simulink model "Coupled_Model_V2_C"  (R2024b)
settings: Solver=FixedStepAuto  StartTime=0.0  StopTime=20  FixedStep=0.001  RelTol=1e-3
values from neighbouring files (symbols this model uses):
  A = 2    [Setup_script_coupled_v1.m]    (also in animation_coupled_model.m; wheel_velocity_demonstrations.m)
  a = 0.8    [Setup_script_coupled_v1.m]    (also in animation_coupled_model.m; wheel_velocity_demonstrations.m)
  b = 1    [Setup_script_coupled_v1.m]    (also in animation_coupled_model.m; wheel_velocity_demonstrations.m)
  brake_bias = 0.5    [Setup_script_coupled_v1.m]    (also in animation_coupled_model.m; wheel_velocity_demonstrations.m)
  brake_torque = [0, 25, 50, 100, 125, 150, 175, 200]    [Setup_script_coupled_v1.m]    (also in animation_coupled_model.m; wheel_velocity_demonstrations.m)
  c = 0.8    [Setup_script_coupled_v1.m]    (also in animation_coupled_model.m; wheel_velocity_demonstrations.m)
  c_alpha = 30000    [Setup_script_coupled_v1.m]    (also in animation_coupled_model.m; wheel_velocity_demonstrations.m)
  C_d = 0.3    [Setup_script_coupled_v1.m]    (also in animation_coupled_model.m; wheel_velocity_demonstrations.m)
  c_sigma = 8000    [Setup_script_coupled_v1.m]    (also in animation_coupled_model.m; wheel_velocity_demonstrations.m)
  d = 0.5    [Setup_script_coupled_v1.m]    (also in animation_coupled_model.m; wheel_velocity_demonstrations.m)
  drivetrain_e = 0.8    [Setup_script_coupled_v1.m]    (also in animation_coupled_model.m; wheel_velocity_demonstrations.m)
  e = 1    [Setup_script_coupled_v1.m]    (also in animation_coupled_model.m; wheel_velocity_demonstrations.m)
  F_i_r = m_i*g-F_h    (= 327)    [Setup_script_coupled_v1.m]    (also in animation_coupled_model.m; wheel_velocity_demonstrations.m)
  F_t_f = (m_t*g*b - F_h*c)/(a+b)    (= 1889.33333333)    [Setup_script_coupled_v1.m]    (also in animation_coupled_model.m; wheel_velocity_demonstrations.m)
  F_t_r = (m_t*g*a + F_h*(b+a))/(a+b)    (= 2398)    [Setup_script_coupled_v1.m]    (also in animation_coupled_model.m; wheel_velocity_demonstrations.m)
  gr = 1    [Setup_script_coupled_v1.m]    (also in animation_coupled_model.m; wheel_velocity_demonstrations.m)
  I_pin = Izz_i + m_i*(d^2)    (= 525)    [Setup_script_coupled_v1.m]    (also in animation_coupled_model.m; wheel_velocity_demonstrations.m)
  I_wheel = 20    [Setup_script_coupled_v1.m]    (also in animation_coupled_model.m; wheel_velocity_demonstrations.m)
  Izz_t = 1000    [Setup_script_coupled_v1.m]    (also in animation_coupled_model.m; wheel_velocity_demonstrations.m)
  m_i = 100    [Setup_script_coupled_v1.m]    (also in animation_coupled_model.m; wheel_velocity_demonstrations.m)
  m_t = 400    [Setup_script_coupled_v1.m]    (also in animation_coupled_model.m; wheel_velocity_demonstrations.m)
  mu = 0.7    [Setup_script_coupled_v1.m]    (also in animation_coupled_model.m; wheel_velocity_demonstrations.m)
  peak_slip = 14*(pi/180)    (= 0.244346095279)    [Setup_script_coupled_v1.m]    (also in animation_coupled_model.m; wheel_velocity_demonstrations.m)
  r = 0.5    [Setup_script_coupled_v1.m]    (also in animation_coupled_model.m = 0.25; wheel_velocity_demonstrations.m)
  rear_braking = 0.3    [Setup_script_coupled_v1.m]    (also in animation_coupled_model.m; wheel_velocity_demonstrations.m)
  rho = 1.225    [Setup_script_coupled_v1.m]    (also in animation_coupled_model.m; wheel_velocity_demonstrations.m)
  slip_coeff = 0.3    [Setup_script_coupled_v1.m]    (also in animation_coupled_model.m; wheel_velocity_demonstrations.m)
  torque_curve = [200, 225, 300, 400, 500, 400, 350, 300, 250, 200]    [Setup_script_coupled_v1.m]    (also in animation_coupled_model.m; wheel_velocity_demonstrations.m)
  torque_omega = linspace(0, 100, length(torque_curve))    [Setup_script_coupled_v1.m]    (also in animation_coupled_model.m; wheel_velocity_demonstrations.m)
libraries: simulink x6
settings Model: Creator=lucas  LastModifiedBy=lucas
settings RTWCC: GPUComputeCapability=3.5

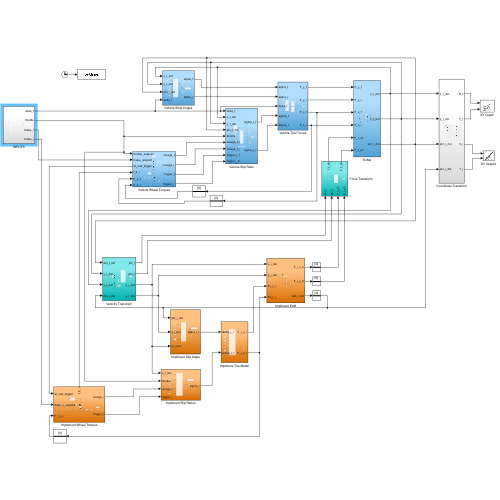
[thumbnail: Simulink's stored preview of the top-level diagram]
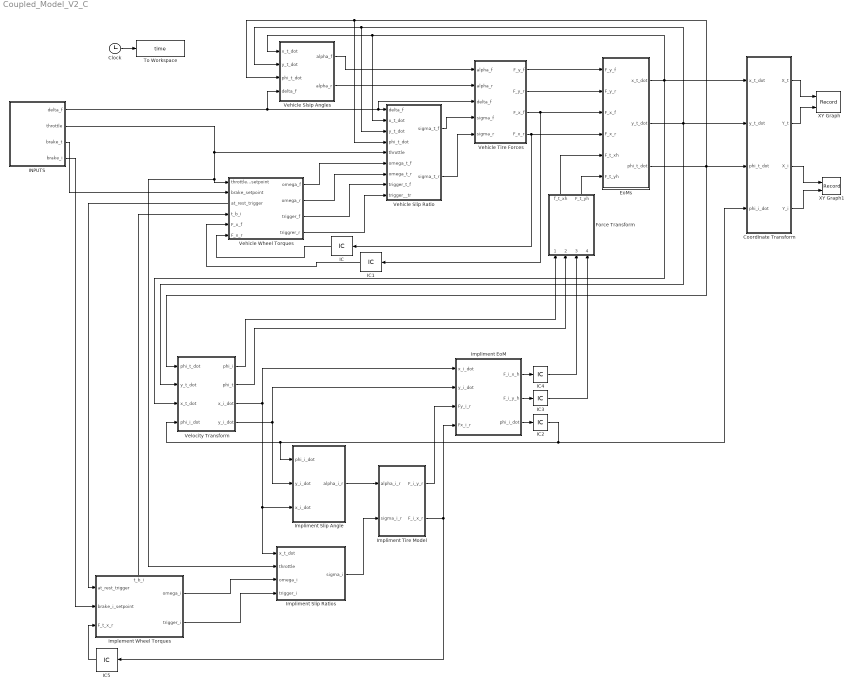
== system Coupled_Model_V2_C ==
  Clock : Clock
  Coordinate Transform : Subsystem
  EoMs : Subsystem
  Force Transform : Subsystem
  IC{,1..5} (6 alike) : InitialCondition  Value=0
  INPUTS : Subsystem
  Implement Wheel Torques : Subsystem
      settings: PortSchema="{\"entries\":[{\"content\":{\"sides\":[{\"content\":{\"connectorIds\":[\"In1\",\"In2\",\"In3\"]},\"type\":\"ConnectorPlacement.EquallySpacedRectSide\",\"uuid\":\"bbf6a9be-76e8-462d-8c03-7de9f71c826e\"},{\"content\":{\"connectorIds\":[\"Out1\",\"Out2\"],\"side\":\"RIGHT\"},\"type\":\"ConnectorPlacement.EquallySpacedRectSide\",\"uuid\":\"22c72d93-0b71-491c-9577-8b76a7679b09\"},{\"content\":{\"connectorIds\":[\"Out3\"],\"side\":\"TOP\"},\"type\":\"ConnectorPlacement.EquallySpacedRectSide\",\"uuid\":\"45839a72-84ef-4b1f-bdc9-287e587f29dc\"}]},\"type\":\"ConnectorPlacement.EquallySpacedConnector\",\"uuid\":\"4d5f4a3e-e594-4f83-8ae5-26ac09bc8c03\"}],\"packageUris\":[\"http://schema.mathworks.com/mf0/Connector/R2020b\"],\"version\":\"1.0\"}"
  Impliment EoM : Subsystem
  Impliment Slip Angle : Subsystem
  Impliment Slip Ratios : Subsystem
  Impliment Tire Model : Subsystem
  To Workspace : ToWorkspace  VariableName=time  SampleTime=-1
  Vehicle Slip Ratio : Subsystem
  Vehicle Slsip Angles : Subsystem
  Vehicle Tire Forces : Subsystem
  Vehicle Wheel Torques : Subsystem
      settings: PortSchema="{\"entries\":[{\"content\":{\"sides\":[{\"content\":{\"connectorIds\":[\"In1\",\"In2\",\"Out5\",\"In3\",\"In4\",\"In5\"]},\"type\":\"ConnectorPlacement.EquallySpacedRectSide\",\"uuid\":\"97f0ad85-6ca5-45e3-95d7-3162af9512d0\"},{\"content\":{\"connectorIds\":[\"Out1\",\"Out2\",\"Out3\",\"Out4\"],\"side\":\"RIGHT\"},\"type\":\"ConnectorPlacement.EquallySpacedRectSide\",\"uuid\":\"abd0d406-3846-4e2f-a2bd-cc2469c5c0c0\"},{\"content\":{\"side\":\"TOP\"},\"type\":\"ConnectorPlacement.EquallySpacedRectSide\",\"uuid\":\"f01a65c6-04bb-49b6-b263-3135f7c7baf2\"},{\"content\":{\"side\":\"BOTTOM\"},\"type\":\"ConnectorPlacement.EquallySpacedRectSide\",\"uuid\":\"a043eba9-81df-4422-b100-d3d245de4c1f\"}]},\"type\":\"ConnectorPlacement.EquallySpacedConnector\",\"uuid\":\"70439dd4-304f-4f7f-8815-0958974c2433\"}],\"packageUris\":[\"http://schema.mathworks.com/mf0/Connector/R2020b\"],\"version\":\"1.0\"}"
  Velocity Transform : Subsystem
  XY Graph : Record  FileSettingsInternal="{\"entries\":[{\"content\":{\"excelSettings\":{\"content\":{},\"type\":\"Streamout.ExcelSettings\"}},\"type\":\"Streamout.FileSettingStorage\",\"uuid\":\"\"}],\"packageUris\":[\"http:\\/\\/schema.mathworks.com\\/mf0\\/streamout_blocks\\/R2020a\"],\"version\":\"1.0\"}"  Layout=[1 1]  SignalsInternal="{\"entries\":[{\"content\":{\"signals\":[{\"content\":{\"blockPath\":[],\"dimensions\":[1],\"domain\":\"\",\"lineColor\":\"#139fff\",\"lineWidth\":2,\"port\":1,\"sid\":[\"\"],\"signalID\":1,\"signalName\":\"Coordinate Transform:1\"},\"type\":\"RecordBlkView.Signal\",\"uuid\":\"\"},{\"content\":{\"blockPath\":[],\"dimensions\":[1],\"domain\":\"\",\"lineColor\":\"#ff6929\",\"lineWidth\":2,\"port\":2,\"sid\":[\"\"],\"signalID\":2,\"signalName\":\"Coordinate Transform:2\"},\"type\":\"RecordBlkView.Signal\",\"uuid\":\"\"}]},\"type\":\"RecordBlkView.InputSignals\",\"uuid\":\"\"}],\"packageUris\":[\"http:\\/\\/schema.mathworks.com\\/mf0\\/streamout_blocks\\/R2020a\"],\"version\":\"1.0\"}"  VisualizationBindings="{\"xyplotplugin\":{\"info\":[{\"series\":[],\"subplotID\":1}]}}"  CompatibilityTag=XY
  XY Graph1 : Record  FileSettingsInternal="{\"entries\":[{\"content\":{\"excelSettings\":{\"content\":{},\"type\":\"Streamout.ExcelSettings\"}},\"type\":\"Streamout.FileSettingStorage\",\"uuid\":\"\"}],\"packageUris\":[\"http:\\/\\/schema.mathworks.com\\/mf0\\/streamout_blocks\\/R2020a\"],\"version\":\"1.0\"}"  Layout=[1 1]  SignalsInternal="{\"entries\":[{\"content\":{\"signals\":[{\"content\":{\"blockPath\":[],\"dimensions\":[1],\"domain\":\"\",\"lineColor\":\"#b746ff\",\"lineWidth\":2,\"port\":1,\"sid\":[\"\"],\"signalID\":1,\"signalName\":\"Coordinate Transform:3\"},\"type\":\"RecordBlkView.Signal\",\"uuid\":\"\"},{\"content\":{\"blockPath\":[],\"dimensions\":[1],\"domain\":\"\",\"lineColor\":\"#64d413\",\"lineWidth\":2,\"port\":2,\"sid\":[\"\"],\"signalID\":2,\"signalName\":\"Coordinate Transform:4\"},\"type\":\"RecordBlkView.Signal\",\"uuid\":\"\"}]},\"type\":\"RecordBlkView.InputSignals\",\"uuid\":\"\"}],\"packageUris\":[\"http:\\/\\/schema.mathworks.com\\/mf0\\/streamout_blocks\\/R2020a\"],\"version\":\"1.0\"}"  VisualizationBindings="{\"xyplotplugin\":{\"info\":[{\"series\":[],\"subplotID\":1}]}}"  CompatibilityTag=XY
  wires:
  EoMs/2(y_t_dot) -> Velocity Transform/2(y_t_dot), Coordinate Transform/2(y_t_dot), Vehicle Slip Ratio/3(y_t_dot), Vehicle Slsip Angles/2(y_t_dot)
  Vehicle Slip Ratio/1(sigma_t_f) -> Vehicle Tire Forces/4(sigma_f)
  Vehicle Slip Ratio/2(sigma_t_r) -> Vehicle Tire Forces/5(sigma_r)
  Vehicle Wheel Torques/1(omega_f) -> Vehicle Slip Ratio/6(omega_t_f)
  INPUTS/1(delta_f) -> Vehicle Slsip Angles/4(delta_f), Vehicle Tire Forces/3(delta_f), Vehicle Slip Ratio/1(delta_f)
  EoMs/3(phi_t_dot) -> Velocity Transform/1(phi_t_dot), Vehicle Slip Ratio/4(phi_t_dot), Vehicle Slsip Angles/3(phi_t_dot), Coordinate Transform/3(phi_t_dot)
  Vehicle Wheel Torques/2(omega_r) -> Vehicle Slip Ratio/7(omega_t_r)
  Vehicle Tire Forces/4(F_x_r) -> IC/1, EoMs/4(F_x_r)
  IC/1 -> Vehicle Wheel Torques/5(F_x_r)
  IC1/1 -> Vehicle Wheel Torques/4(F_x_f)
  Vehicle Tire Forces/3(F_x_f) -> IC1/1, EoMs/3(F_x_f)
  EoMs/1(x_t_dot) -> Velocity Transform/3(x_t_dot), Coordinate Transform/1(x_t_dot), Vehicle Slip Ratio/2(x_t_dot), Vehicle Slsip Angles/1(x_t_dot)
  Coordinate Transform/1(X_t) -> XY Graph/1
  Coordinate Transform/2(Y_t) -> XY Graph/2
  INPUTS/3(brake_t) -> Vehicle Wheel Torques/2(brake_setpoint)
  Vehicle Wheel Torques/3(trigger_f) -> Vehicle Slip Ratio/8(trigger_t_f)
  Vehicle Wheel Torques/4(triggrer_r) -> Vehicle Slip Ratio/9(trigger__tr)
  INPUTS/2(throttle) -> Impliment Slip Ratios/2(throttle), Vehicle Wheel Torques/1(throttle_setpoint), Vehicle Slip Ratio/5(throttle)
  Clock/1 -> To Workspace/1
  Velocity Transform/3(x_i_dot) -> Impliment Slip Angle/3(x_i_dot), Impliment Slip Ratios/1(x_t_dot), Impliment EoM/1(x_i_dot)
  Velocity Transform/4(y_i_dot) -> Impliment EoM/2(y_i_dot), Impliment Slip Angle/2(y_i_dot)
  Impliment EoM/3(phi_i_dot) -> IC2/1
  Impliment EoM/1(F_i_x_h) -> IC4/1
  Impliment EoM/2(F_i_y_h) -> IC3/1
  IC3/1 -> Force Transform/4(F_i_yh)
  IC4/1 -> Force Transform/3(F_i_xh)
  IC2/1 -> Coordinate Transform/4(phi_i_dot), Velocity Transform/4(phi_i_dot), Impliment Slip Angle/1(phi_i_dot)
  Coordinate Transform/3(X_i) -> XY Graph1/1
  Coordinate Transform/4(Y_i) -> XY Graph1/2
  Impliment Tire Model/1(F_i_y_r) -> Impliment EoM/3(Fy_i_r)
  Impliment Tire Model/2(F_i_x_r) -> IC5/1, Impliment EoM/4(Fx_i_r)
  Impliment Slip Ratios/1(sigma_i) -> Impliment Tire Model/2(sigma_i_r)
  Force Transform/2(F_t_yh) -> EoMs/6(F_t_yh)
  Force Transform/1(f_t_xh) -> EoMs/5(F_t_xh)
  Velocity Transform/2(phi_t) -> Force Transform/2(phi_t)
  Velocity Transform/1(phi_i) -> Force Transform/1(phi_i)
  Implement Wheel Torques/1(omega_i) -> Impliment Slip Ratios/3(omega_i)
  Implement Wheel Torques/2(trigger_i) -> Impliment Slip Ratios/4(trigger_i)
  Implement Wheel Torques/3(t_b_i) -> Vehicle Wheel Torques/3(t_b_i)
  INPUTS/4(brake_i) -> Implement Wheel Torques/2(brake_i_setpoint)
  IC5/1 -> Implement Wheel Torques/3(F_t_x_r)
  Vehicle Wheel Torques/5(at_rest_trigger) -> Implement Wheel Torques/1(at_rest_trigger)
  Vehicle Slsip Angles/2(alpha_r) -> Vehicle Tire Forces/2(alpha_r)
  Vehicle Slsip Angles/1(alpha_f) -> Vehicle Tire Forces/1(alpha_f)
  Vehicle Tire Forces/1(F_y_f) -> EoMs/1(F_y_f)
  Vehicle Tire Forces/2(F_y_r) -> EoMs/2(F_y_r)
  Impliment Slip Angle/1(alpha_i_r) -> Impliment Tire Model/1(alpha_i_r)

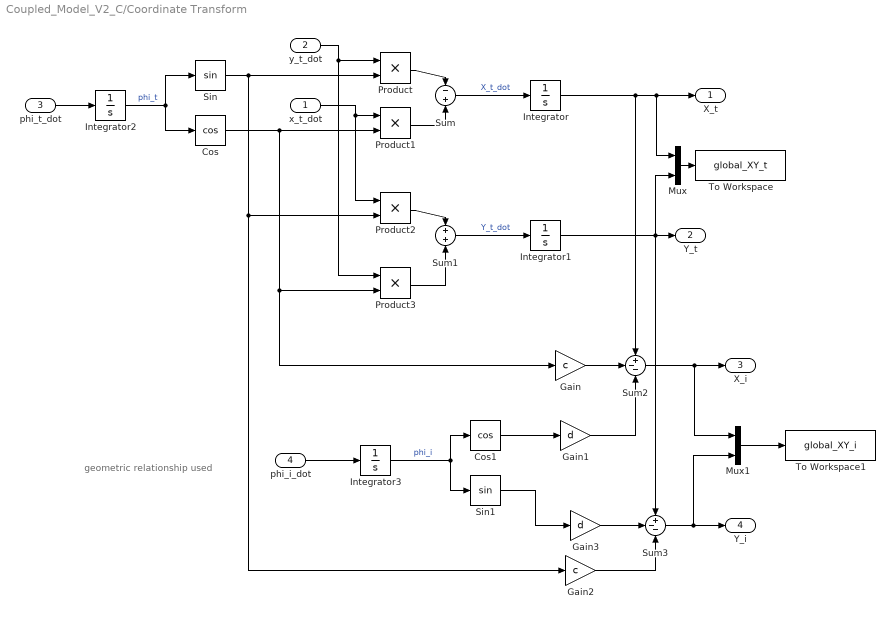
== system Coupled_Model_V2_C/Coordinate Transform ==
  note: geometric relationship used
  x_t_dot : Inport
  y_t_dot : Inport  Port=2
  phi_t_dot : Inport  Port=3
  phi_i_dot : Inport  Port=4
  Cos : Trigonometry  Operator=cos
  Cos1 : Trigonometry  Operator=cos
  Gain : Gain  Gain=c
  Gain1 : Gain  Gain=d
  Gain2 : Gain  Gain=c
  Gain3 : Gain  Gain=d
  Integrator{,1..3} (4 alike) : Integrator
  Mux : Mux  Inputs=2
  Mux1 : Mux  Inputs=2
  Product{,1..3} (4 alike) : Product
  Sin : Trigonometry
  Sin1 : Trigonometry
  Sum : Sum  Inputs=-+
  Sum1 : Sum
  Sum2 : Sum  Inputs=+--
  Sum3 : Sum  Inputs=+--
  To Workspace : ToWorkspace  VariableName=global_XY_t  SampleTime=-1
  To Workspace1 : ToWorkspace  VariableName=global_XY_i  SampleTime=-1
  X_t : Outport
  Y_t : Outport  Port=2
  X_i : Outport  Port=3
  Y_i : Outport  Port=4
  wires:
  Integrator/1 -> Sum2/1, Mux/1, X_t/1
  Integrator1/1 -> Mux/2, Y_t/1, Sum3/1
  Sum/1 -> Integrator/1  "X_t_dot"
  Sum1/1 -> Integrator1/1  "Y_t_dot"
  Sin/1 -> Product/2, Gain2/1, Product2/2
  Product/1 -> Sum/1
  Product1/1 -> Sum/2
  y_t_dot/1 -> Product/1, Product3/1
  Product2/1 -> Sum1/1
  Product3/1 -> Sum1/2
  Cos/1 -> Gain/1, Product3/2, Product1/2
  x_t_dot/1 -> Product1/1, Product2/1
  phi_t_dot/1 -> Integrator2/1
  Integrator2/1 -> Sin/1, Cos/1  "phi_t"
  Mux/1 -> To Workspace/1
  phi_i_dot/1 -> Integrator3/1
  Integrator3/1 -> Cos1/1, Sin1/1  "phi_i"
  Gain/1 -> Sum2/2
  Gain1/1 -> Sum2/3
  Cos1/1 -> Gain1/1
  Sum3/1 -> Mux1/2, Y_i/1
  Gain2/1 -> Sum3/3
  Gain3/1 -> Sum3/2
  Sin1/1 -> Gain3/1
  Mux1/1 -> To Workspace1/1
  Sum2/1 -> Mux1/1, X_i/1

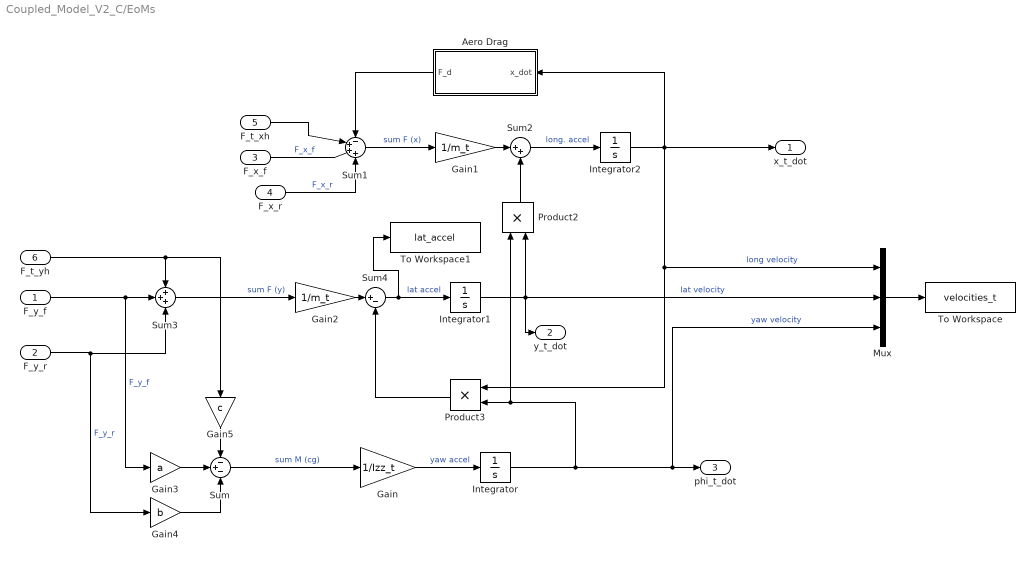
== system Coupled_Model_V2_C/EoMs ==
  F_y_f : Inport
  F_y_r : Inport  Port=2
  F_x_f : Inport  Port=3
  F_x_r : Inport  Port=4
  F_t_xh : Inport  Port=5
  F_t_yh : Inport  Port=6
  Aero Drag : Subsystem
  Gain : Gain  Gain=1/Izz_t
  Gain1 : Gain  Gain=1/m_t
  Gain2 : Gain  Gain=1/m_t
  Gain3 : Gain  Gain=a
  Gain4 : Gain  Gain=b
  Gain5 : Gain  Gain=c
  Integrator : Integrator
  Integrator1 : Integrator
  Integrator2 : Integrator
  Mux : Mux  Inputs=3
  Product2 : Product
  Product3 : Product
  Sum : Sum  Inputs=-+-
  Sum1 : Sum  Inputs=-+++
  Sum2 : Sum  Inputs=|++
  Sum3 : Sum  Inputs=+++
  Sum4 : Sum  Inputs=|+-
  To Workspace : ToWorkspace  VariableName=velocities_t  SampleTime=-1
  To Workspace1 : ToWorkspace  VariableName=lat_accel  SampleTime=-1
  x_t_dot : Outport
  y_t_dot : Outport  Port=2
  phi_t_dot : Outport  Port=3
  wires:
  Integrator1/1 -> Product2/2, Mux/2, y_t_dot/1  "lat velocity"
  Sum4/1 -> To Workspace1/1, Integrator1/1  "lat accel"
  F_y_r/1 -> Sum3/3, Gain4/1  "F_y_r"
  Sum3/1 -> Gain2/1  "sum F (y)"
  Product3/1 -> Sum4/2
  Sum/1 -> Gain/1  "sum M (cg)"
  Gain/1 -> Integrator/1  "yaw accel"
  Product2/1 -> Sum2/2
  Gain2/1 -> Sum4/1
  Gain1/1 -> Sum2/1
  Integrator/1 -> Mux/3, phi_t_dot/1, Product3/2, Product2/1  "yaw velocity"
  F_y_f/1 -> Sum3/2, Gain3/1  "F_y_f"
  Sum1/1 -> Gain1/1  "sum F (x)"
  Sum2/1 -> Integrator2/1  "long. accel"
  Integrator2/1 -> x_t_dot/1, Aero Drag/1(x_dot), Product3/1, Mux/1  "long velocity"
  Aero Drag/1(F_d) -> Sum1/1
  Mux/1 -> To Workspace/1
  Gain4/1 -> Sum/3
  Gain3/1 -> Sum/2
  Gain5/1 -> Sum/1
  F_x_r/1 -> Sum1/4  "F_x_r"
  F_x_f/1 -> Sum1/3  "F_x_f"
  F_t_xh/1 -> Sum1/2
  F_t_yh/1 -> Gain5/1, Sum3/1

== system Coupled_Model_V2_C/Force Transform ==
  phi_i : Inport
  phi_t : Inport  Port=2
  F_i_xh : Inport  Port=3
  F_i_yh : Inport  Port=4
  MATLAB Function : MATLAB Function  TreatAsAtomicUnit=on
  Mux : Mux  Inputs=2
  To Workspace : ToWorkspace  VariableName=coupling_force  SampleTime=-1
  f_t_xh : Outport
  F_t_yh : Outport  Port=2
  wires:
  phi_i/1 -> MATLAB Function/1(phi_i)
  phi_t/1 -> MATLAB Function/2(phi_t)
  F_i_xh/1 -> MATLAB Function/3(F_i_xh)
  F_i_yh/1 -> MATLAB Function/4(F_i_yh)
  MATLAB Function/1(F_t_x) -> Mux/1, f_t_xh/1
  MATLAB Function/2(F_t_y) -> Mux/2, F_t_yh/1
  Mux/1 -> To Workspace/1

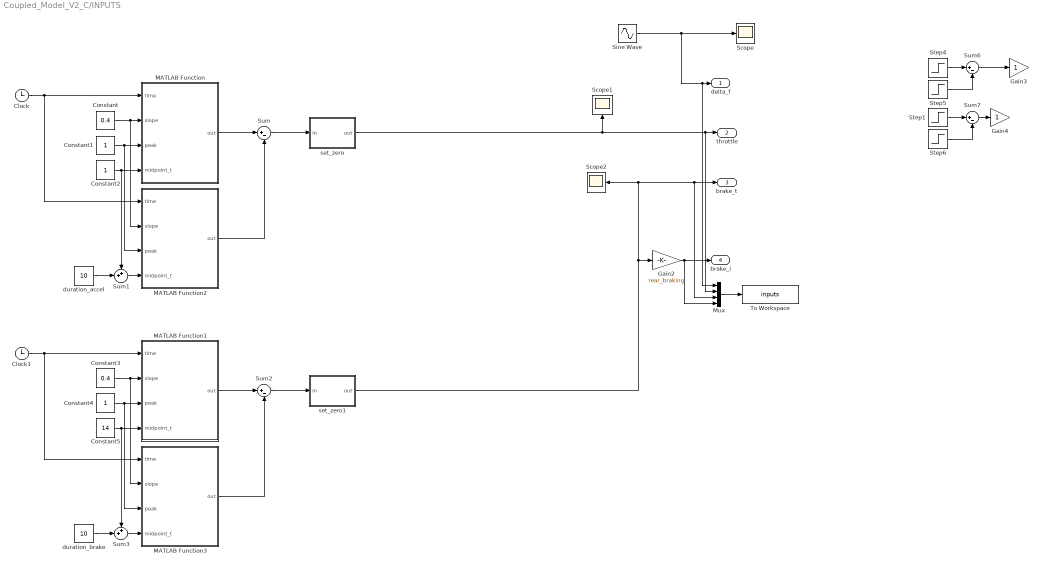
== system Coupled_Model_V2_C/INPUTS ==
  Clock : Clock
  Clock1 : Clock
  Constant : Constant  Value=0.4
  Constant1 : Constant
  Constant2 : Constant
  Constant3 : Constant  Value=0.4
  Constant4 : Constant
  Constant5 : Constant  Value=14
  Gain2 : Gain  Gain=rear_braking
  Gain3 : Gain
  Gain4 : Gain
  MATLAB Function : MATLAB Function  TreatAsAtomicUnit=on
  MATLAB Function1 : MATLAB Function  TreatAsAtomicUnit=on
  MATLAB Function2 : MATLAB Function  TreatAsAtomicUnit=on
  MATLAB Function3 : MATLAB Function  TreatAsAtomicUnit=on
  Mux : Mux
  Scope : Scope
  Scope1 : Scope
  Scope2 : Scope
  Sine Wave : Sin  Amplitude=0.2  Frequency=0.5  SampleTime=0
  Step1 : Step  Time=14  SampleTime=0
  Step4 : Step  SampleTime=0
  Step5 : Step  Time=13  SampleTime=0
  Step6 : Step  Time=20  SampleTime=0
  Sum{,2,6..7} (4 alike) : Sum  Inputs=|+-
  Sum1 : Sum  Inputs=++|
  Sum3 : Sum  Inputs=++|
  To Workspace : ToWorkspace  VariableName=inputs  SampleTime=-1
  duration_accel : Constant  Value=10
  duration_brake : Constant  Value=10
  set_zero : MATLAB Function  TreatAsAtomicUnit=on
  set_zero1 : MATLAB Function  TreatAsAtomicUnit=on
  delta_f : Outport
  throttle : Outport  Port=2
  brake_t : Outport  Port=3
  brake_i : Outport  Port=4
  wires:
  Sine Wave/1 -> Mux/1, delta_f/1, Scope/1
  Mux/1 -> To Workspace/1
  Gain2/1 -> Mux/4, brake_i/1
  set_zero/1(out) -> throttle/1, Mux/2, Scope1/1
  set_zero1/1(out) -> Scope2/1, Mux/3, brake_t/1, Gain2/1
  Sum6/1 -> Gain3/1
  Step5/1 -> Sum6/2
  Step4/1 -> Sum6/1
  Step6/1 -> Sum7/2
  Sum7/1 -> Gain4/1
  Step1/1 -> Sum7/1
  Sum1/1 -> MATLAB Function2/4(midpoint_t)
  Constant2/1 -> Sum1/1, MATLAB Function/4(midpoint_t)
  Sum/1 -> set_zero/1(in)
  Constant/1 -> MATLAB Function2/2(slope), MATLAB Function/2(slope)
  duration_accel/1 -> Sum1/2
  Constant1/1 -> MATLAB Function2/3(peak), MATLAB Function/3(peak)
  MATLAB Function2/1(out) -> Sum/2
  Clock/1 -> MATLAB Function2/1(time), MATLAB Function/1(time)
  MATLAB Function/1(out) -> Sum/1
  MATLAB Function1/1(out) -> Sum2/1
  MATLAB Function3/1(out) -> Sum2/2
  Clock1/1 -> MATLAB Function3/1(time), MATLAB Function1/1(time)
  Constant3/1 -> MATLAB Function3/2(slope), MATLAB Function1/2(slope)
  duration_brake/1 -> Sum3/2
  Sum3/1 -> MATLAB Function3/4(midpoint_t)
  Sum2/1 -> set_zero1/1(in)
  Constant4/1 -> MATLAB Function3/3(peak), MATLAB Function1/3(peak)
  Constant5/1 -> Sum3/1, MATLAB Function1/4(midpoint_t)

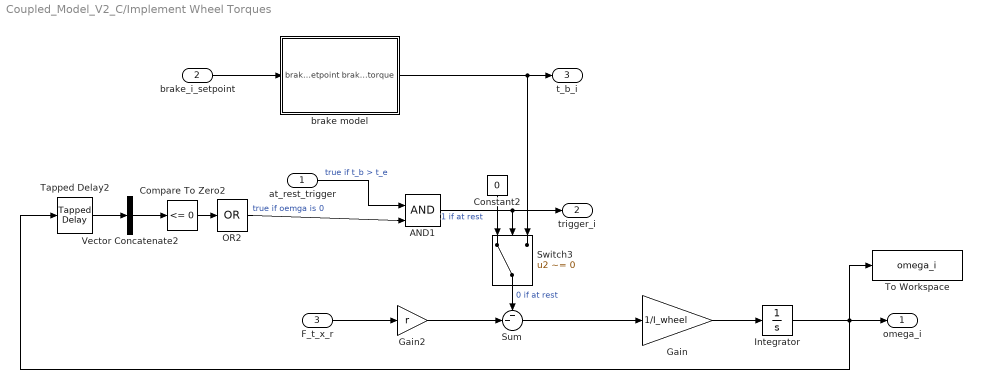
== system Coupled_Model_V2_C/Implement Wheel Torques ==
  at_rest_trigger : Inport
  brake_i_setpoint : Inport  Port=2
  F_t_x_r : Inport  Port=3
  AND1 : Logic  IconShape=distinctive  AllPortsSameDT=off  OutDataTypeStr=boolean
  Compare To Zero2 : simulink/Logic and Bit Operations/Compare To Zero  relop=<=  OutDataTypeStr=boolean
  Constant2 : Constant  Value=0
  Gain : Gain  Gain=1/I_wheel
  Gain2 : Gain  Gain=r
  Integrator : Integrator
  OR2 : Logic  Operator=OR  Inputs=1  IconShape=distinctive  AllPortsSameDT=off  OutDataTypeStr=boolean
  Sum : Sum  Inputs=--|
  Switch3 : Switch  Criteria=u2 ~= 0  SaturateOnIntegerOverflow=off  InputSameDT=off
  Tapped Delay2 : simulink/Discrete/Tapped Delay  vinit=0.0  samptime=-1  NumDelays=20  DelayOrder=Oldest  includeCurrent=off
  To Workspace : ToWorkspace  VariableName=omega_i  SampleTime=-1
  Vector Concatenate2 : Concatenate  NumInputs=1
  brake model : Subsystem
  omega_i : Outport
  trigger_i : Outport  Port=2
  t_b_i : Outport  Port=3
  wires:
  brake_i_setpoint/1 -> brake model/1(brake_setpoint)
  Gain/1 -> Integrator/1
  Sum/1 -> Gain/1
  F_t_x_r/1 -> Gain2/1
  Gain2/1 -> Sum/2
  Constant2/1 -> Switch3/1
  brake model/1(brake_torque) -> t_b_i/1, Switch3/3
  Switch3/1 -> Sum/1  "0 if at rest"
  AND1/1 -> trigger_i/1, Switch3/2  "1 if at rest"
  Tapped Delay2/1 -> Vector Concatenate2/1
  Vector Concatenate2/1 -> Compare To Zero2/1
  Compare To Zero2/1 -> OR2/1
  OR2/1 -> AND1/2  "true if oemga is 0"
  Integrator/1 -> To Workspace/1, Tapped Delay2/1, omega_i/1
  at_rest_trigger/1 -> AND1/1  "true if t_b > t_e"

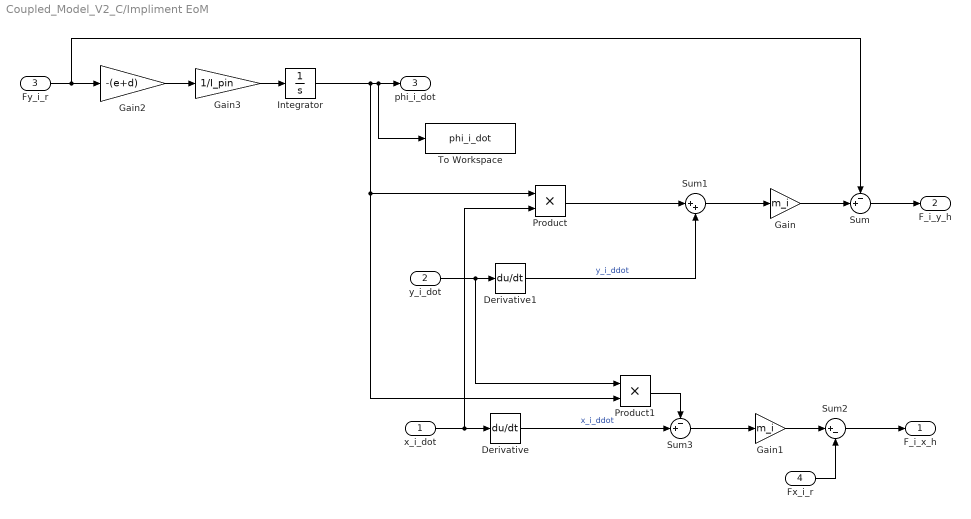
== system Coupled_Model_V2_C/Impliment EoM ==
  x_i_dot : Inport
  y_i_dot : Inport  Port=2
  Fy_i_r : Inport  Port=3
  Fx_i_r : Inport  Port=4
  Derivative : Derivative
  Derivative1 : Derivative
  Gain : Gain  Gain=m_i
  Gain1 : Gain  Gain=m_i
  Gain2 : Gain  Gain=-(e+d)
  Gain3 : Gain  Gain=1/I_pin
  Integrator : Integrator
  Product : Product
  Product1 : Product
  Sum : Sum  Inputs=-+|
  Sum1 : Sum  Inputs=|++
  Sum2 : Sum  Inputs=|+-
  Sum3 : Sum  Inputs=-+|
  To Workspace : ToWorkspace  VariableName=phi_i_dot  SampleTime=-1
  F_i_x_h : Outport
  F_i_y_h : Outport  Port=2
  phi_i_dot : Outport  Port=3
  wires:
  x_i_dot/1 -> Product/2, Derivative/1
  y_i_dot/1 -> Product1/1, Derivative1/1
  Derivative1/1 -> Sum1/2  "y_i_ddot"
  Sum/1 -> F_i_y_h/1
  Gain/1 -> Sum/2
  Sum1/1 -> Gain/1
  Integrator/1 -> To Workspace/1, phi_i_dot/1, Product/1, Product1/2
  Product/1 -> Sum1/1
  Sum2/1 -> F_i_x_h/1
  Fx_i_r/1 -> Sum2/2
  Gain1/1 -> Sum2/1
  Sum3/1 -> Gain1/1
  Derivative/1 -> Sum3/2  "x_i_ddot"
  Product1/1 -> Sum3/1
  Fy_i_r/1 -> Sum/1, Gain2/1
  Gain2/1 -> Gain3/1
  Gain3/1 -> Integrator/1

== system Coupled_Model_V2_C/Impliment Slip Angle ==
  phi_i_dot : Inport
  y_i_dot : Inport  Port=2
  x_i_dot : Inport  Port=3
  Constant : Constant  Value=e
  MATLAB Function : MATLAB Function  TreatAsAtomicUnit=on
  To Workspace : ToWorkspace  VariableName=slip_angles_i  SampleTime=-1
  alpha_i_r : Outport
  wires:
  y_i_dot/1 -> MATLAB Function/1(y_dot)
  x_i_dot/1 -> MATLAB Function/2(x_dot)
  phi_i_dot/1 -> MATLAB Function/3(phi_dot)
  Constant/1 -> MATLAB Function/4(e)
  MATLAB Function/1(alpha) -> To Workspace/1, alpha_i_r/1

== system Coupled_Model_V2_C/Impliment Slip Ratios ==
  x_t_dot : Inport
  throttle : Inport  Port=2
  omega_i : Inport  Port=3
  trigger_i : Inport  Port=4
  Constant : Constant  Value=r
  To Workspace : ToWorkspace  VariableName=sigma_i  SampleTime=-1
  slip_ratio : MATLAB Function  TreatAsAtomicUnit=on
  sigma_i : Outport
  wires:
  x_t_dot/1 -> slip_ratio/1(x_t_dot)
  Constant/1 -> slip_ratio/2(r)
  trigger_i/1 -> slip_ratio/5(trigger)
  throttle/1 -> slip_ratio/4(throttle)
  omega_i/1 -> slip_ratio/3(omega)
  slip_ratio/1(sigma) -> To Workspace/1, sigma_i/1  "front sip ratio"

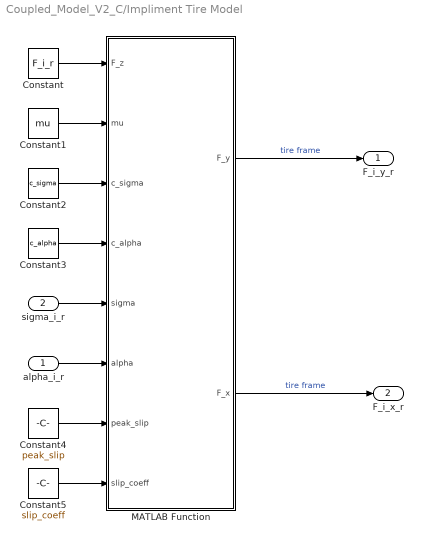
== system Coupled_Model_V2_C/Impliment Tire Model ==
  alpha_i_r : Inport
  sigma_i_r : Inport  Port=2
  Constant : Constant  Value=F_i_r
  Constant1 : Constant  Value=mu
  Constant2 : Constant  Value=c_sigma
  Constant3 : Constant  Value=c_alpha
  Constant4 : Constant  Value=peak_slip
  Constant5 : Constant  Value=slip_coeff
  MATLAB Function : MATLAB Function  TreatAsAtomicUnit=on
  F_i_y_r : Outport
  F_i_x_r : Outport  Port=2
  wires:
  Constant/1 -> MATLAB Function/1(F_z)
  Constant1/1 -> MATLAB Function/2(mu)
  Constant3/1 -> MATLAB Function/4(c_alpha)
  Constant2/1 -> MATLAB Function/3(c_sigma)
  sigma_i_r/1 -> MATLAB Function/5(sigma)
  alpha_i_r/1 -> MATLAB Function/6(alpha)
  MATLAB Function/1(F_y) -> F_i_y_r/1  "tire frame"
  MATLAB Function/2(F_x) -> F_i_x_r/1  "tire frame"
  Constant4/1 -> MATLAB Function/7(peak_slip)
  Constant5/1 -> MATLAB Function/8(slip_coeff)

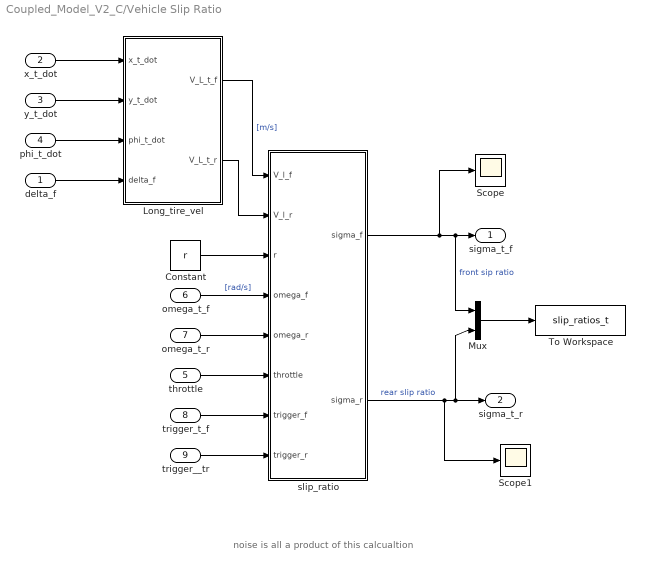
== system Coupled_Model_V2_C/Vehicle Slip Ratio ==
  note: noise is all a product of this calcualtion
  delta_f : Inport
  x_t_dot : Inport  Port=2
  y_t_dot : Inport  Port=3
  phi_t_dot : Inport  Port=4
  throttle : Inport  Port=5
  omega_t_f : Inport  Port=6
  omega_t_r : Inport  Port=7
  trigger_t_f : Inport  Port=8
  trigger__tr : Inport  Port=9
  Constant : Constant  Value=r
  Long_tire_vel : Subsystem
  Mux : Mux  Inputs=2
  Scope : Scope
  Scope1 : Scope
  To Workspace : ToWorkspace  VariableName=slip_ratios_t  SampleTime=-1
  slip_ratio : MATLAB Function  TreatAsAtomicUnit=on
  sigma_t_f : Outport
  sigma_t_r : Outport  Port=2
  wires:
  omega_t_f/1 -> slip_ratio/4(omega_f)  "[rad/s]"
  omega_t_r/1 -> slip_ratio/5(omega_r)
  Long_tire_vel/1(V_L_t_f) -> slip_ratio/1(V_l_f)  "[m/s]"
  Constant/1 -> slip_ratio/3(r)
  slip_ratio/1(sigma_f) -> Scope/1, Mux/1, sigma_t_f/1  "front sip ratio"
  slip_ratio/2(sigma_r) -> Scope1/1, Mux/2, sigma_t_r/1  "rear slip ratio"
  x_t_dot/1 -> Long_tire_vel/1(x_t_dot)
  y_t_dot/1 -> Long_tire_vel/2(y_t_dot)
  phi_t_dot/1 -> Long_tire_vel/3(phi_t_dot)
  delta_f/1 -> Long_tire_vel/4(delta_f)
  Long_tire_vel/2(V_L_t_r) -> slip_ratio/2(V_l_r)
  throttle/1 -> slip_ratio/6(throttle)
  trigger_t_f/1 -> slip_ratio/7(trigger_f)
  trigger__tr/1 -> slip_ratio/8(trigger_r)
  Mux/1 -> To Workspace/1

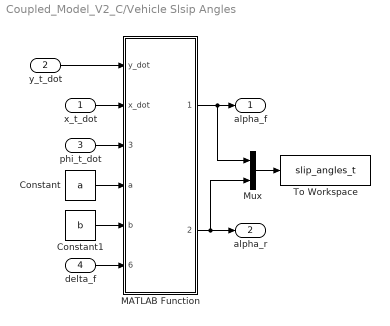
== system Coupled_Model_V2_C/Vehicle Slsip Angles ==
  x_t_dot : Inport
  y_t_dot : Inport  Port=2
  phi_t_dot : Inport  Port=3
  delta_f : Inport  Port=4
  Constant : Constant  Value=a
  Constant1 : Constant  Value=b
  MATLAB Function : MATLAB Function  TreatAsAtomicUnit=on
  Mux : Mux  Inputs=2
  To Workspace : ToWorkspace  VariableName=slip_angles_t  SampleTime=-1
  alpha_f : Outport
  alpha_r : Outport  Port=2
  wires:
  MATLAB Function/1(alpha_f) -> Mux/1, alpha_f/1
  MATLAB Function/2(alpha_r) -> Mux/2, alpha_r/1
  delta_f/1 -> MATLAB Function/6(delta_f)
  phi_t_dot/1 -> MATLAB Function/3(phi_dot)
  x_t_dot/1 -> MATLAB Function/2(x_dot)
  y_t_dot/1 -> MATLAB Function/1(y_dot)
  Constant/1 -> MATLAB Function/4(a)
  Constant1/1 -> MATLAB Function/5(b)
  Mux/1 -> To Workspace/1

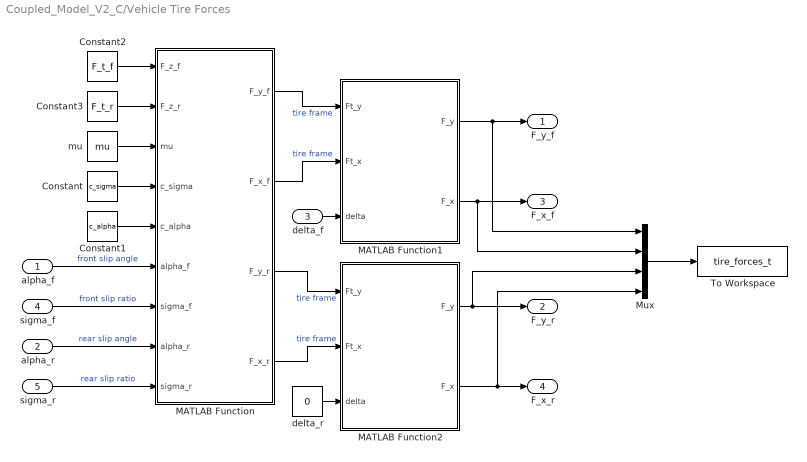
== system Coupled_Model_V2_C/Vehicle Tire Forces ==
  alpha_f : Inport
  alpha_r : Inport  Port=2
  delta_f : Inport  Port=3
  sigma_f : Inport  Port=4
  sigma_r : Inport  Port=5
  Constant : Constant  Value=c_sigma
  Constant1 : Constant  Value=c_alpha
  Constant2 : Constant  Value=F_t_f
  Constant3 : Constant  Value=F_t_r
  MATLAB Function : MATLAB Function  TreatAsAtomicUnit=on
  MATLAB Function1 : MATLAB Function  TreatAsAtomicUnit=on
  MATLAB Function2 : MATLAB Function  TreatAsAtomicUnit=on
  Mux : Mux
  To Workspace : ToWorkspace  VariableName=tire_forces_t  SampleTime=-1
  delta_r : Constant  Value=0
  mu : Constant  Value=mu
  F_y_f : Outport
  F_y_r : Outport  Port=2
  F_x_f : Outport  Port=3
  F_x_r : Outport  Port=4
  wires:
  alpha_f/1 -> MATLAB Function/6(alpha_f)  "front slip angle"
  Constant2/1 -> MATLAB Function/1(F_z_f)
  Constant3/1 -> MATLAB Function/2(F_z_r)
  mu/1 -> MATLAB Function/3(mu)
  Constant/1 -> MATLAB Function/4(c_sigma)
  Constant1/1 -> MATLAB Function/5(c_alpha)
  alpha_r/1 -> MATLAB Function/8(alpha_r)  "rear slip angle"
  sigma_f/1 -> MATLAB Function/7(sigma_f)  "front slip ratio"
  sigma_r/1 -> MATLAB Function/9(sigma_r)  "rear slip ratio"
  MATLAB Function1/1(F_y) -> Mux/1, F_y_f/1
  MATLAB Function1/2(F_x) -> Mux/2, F_x_f/1
  delta_f/1 -> MATLAB Function1/3(delta)
  MATLAB Function/2(F_x_f) -> MATLAB Function1/2(Ft_x)  "tire frame"
  MATLAB Function/1(F_y_f) -> MATLAB Function1/1(Ft_y)  "tire frame"
  MATLAB Function/3(F_y_r) -> MATLAB Function2/1(Ft_y)  "tire frame"
  MATLAB Function/4(F_x_r) -> MATLAB Function2/2(Ft_x)  "tire frame"
  delta_r/1 -> MATLAB Function2/3(delta)
  MATLAB Function2/2(F_x) -> Mux/4, F_x_r/1
  MATLAB Function2/1(F_y) -> F_y_r/1, Mux/3
  Mux/1 -> To Workspace/1

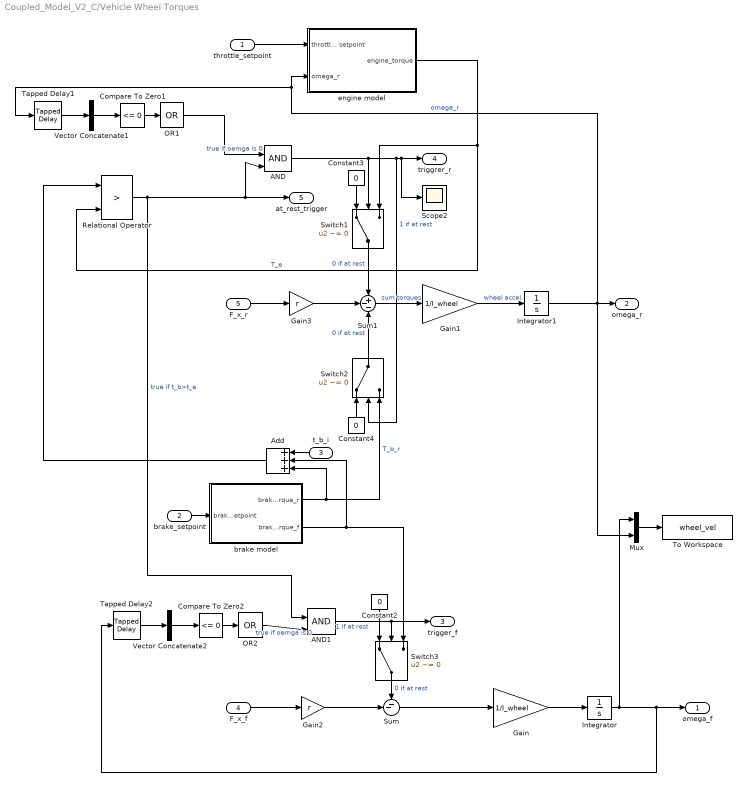
== system Coupled_Model_V2_C/Vehicle Wheel Torques ==
  throttle_setpoint : Inport
  brake_setpoint : Inport  Port=2
  t_b_i : Inport  Port=3
  F_x_f : Inport  Port=4
  F_x_r : Inport  Port=5
  AND : Logic  IconShape=distinctive  AllPortsSameDT=off  OutDataTypeStr=boolean
  AND1 : Logic  IconShape=distinctive  AllPortsSameDT=off  OutDataTypeStr=boolean
  Add : Sum  Inputs=+++
  Compare To Zero1 : simulink/Logic and Bit Operations/Compare To Zero  relop=<=  OutDataTypeStr=boolean
  Compare To Zero2 : simulink/Logic and Bit Operations/Compare To Zero  relop=<=  OutDataTypeStr=boolean
  Constant2 : Constant  Value=0
  Constant3 : Constant  Value=0
  Constant4 : Constant  Value=0
  Gain : Gain  Gain=1/I_wheel
  Gain1 : Gain  Gain=1/I_wheel
  Gain2 : Gain  Gain=r
  Gain3 : Gain  Gain=r
  Integrator : Integrator
  Integrator1 : Integrator
  Mux : Mux  Inputs=2
  OR1 : Logic  Operator=OR  Inputs=1  IconShape=distinctive  AllPortsSameDT=off  OutDataTypeStr=boolean
  OR2 : Logic  Operator=OR  Inputs=1  IconShape=distinctive  AllPortsSameDT=off  OutDataTypeStr=boolean
  Relational Operator : RelationalOperator  Operator=>  OutDataTypeStr=boolean  RndMeth=Simplest  InputSameDT=off
  Scope2 : Scope
  Sum : Sum  Inputs=--|
  Sum1 : Sum  Inputs=+--
  Switch1 : Switch  Criteria=u2 ~= 0  SaturateOnIntegerOverflow=off  InputSameDT=off
  Switch2 : Switch  Criteria=u2 ~= 0  SaturateOnIntegerOverflow=off  InputSameDT=off
  Switch3 : Switch  Criteria=u2 ~= 0  SaturateOnIntegerOverflow=off  InputSameDT=off
  Tapped Delay1 : simulink/Discrete/Tapped Delay  vinit=0.0  samptime=-1  NumDelays=20  DelayOrder=Oldest  includeCurrent=off
  Tapped Delay2 : simulink/Discrete/Tapped Delay  vinit=0.0  samptime=-1  NumDelays=20  DelayOrder=Oldest  includeCurrent=off
  To Workspace : ToWorkspace  VariableName=wheel_vel  SampleTime=-1
  Vector Concatenate1 : Concatenate  NumInputs=1
  Vector Concatenate2 : Concatenate  NumInputs=1
  brake model : Subsystem
  engine model : Subsystem
  omega_f : Outport
  omega_r : Outport  Port=2
  trigger_f : Outport  Port=3
  triggrer_r : Outport  Port=4
  at_rest_trigger : Outport  Port=5
  wires:
  throttle_setpoint/1 -> engine model/1(throttle setpoint)
  brake_setpoint/1 -> brake model/1(brake_setpoint)
  Gain/1 -> Integrator/1
  Gain1/1 -> Integrator1/1  "wheel accel."
  Sum1/1 -> Gain1/1  "sum torques"
  Sum/1 -> Gain/1
  F_x_r/1 -> Gain3/1
  F_x_f/1 -> Gain2/1
  Gain3/1 -> Sum1/2
  Gain2/1 -> Sum/2
  brake model/1(brake_torque_r) -> Add/3, Switch2/3  "T_b_r"
  engine model/1(engine_torque) -> Switch1/3, Relational Operator/2  "T_e"
  Relational Operator/1 -> AND/2, at_rest_trigger/1, AND1/1  "true if t_b>t_e"
  Integrator1/1 -> omega_r/1, Mux/2, Tapped Delay1/1, engine model/2(omega_r)  "omega_r"
  AND/1 -> Scope2/1, triggrer_r/1, Switch2/2, Switch1/2  "1 if at rest"
  Switch1/1 -> Sum1/1  "0 if at rest"
  Switch2/1 -> Sum1/3  "0 if at rest"
  Constant4/1 -> Switch2/1
  Constant3/1 -> Switch1/1
  Constant2/1 -> Switch3/1
  brake model/2(brake_torque_f) -> Add/2, Switch3/3
  Switch3/1 -> Sum/1  "0 if at rest"
  AND1/1 -> trigger_f/1, Switch3/2  "1 if at rest"
  Tapped Delay1/1 -> Vector Concatenate1/1
  Compare To Zero1/1 -> OR1/1
  Vector Concatenate1/1 -> Compare To Zero1/1
  OR1/1 -> AND/1  "true if oemga is 0"
  Add/1 -> Relational Operator/1
  Tapped Delay2/1 -> Vector Concatenate2/1
  Vector Concatenate2/1 -> Compare To Zero2/1
  Compare To Zero2/1 -> OR2/1
  OR2/1 -> AND1/2  "true if oemga is 0"
  Integrator/1 -> Mux/1, Tapped Delay2/1, omega_f/1
  Mux/1 -> To Workspace/1
  t_b_i/1 -> Add/1

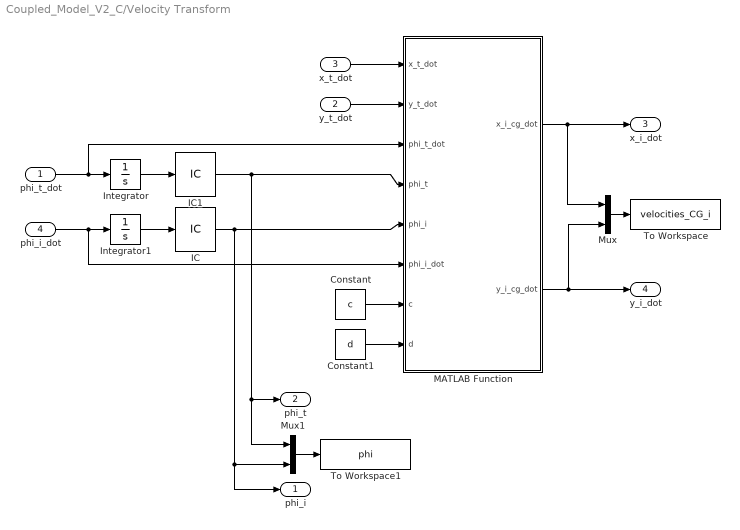
== system Coupled_Model_V2_C/Velocity Transform ==
  phi_t_dot : Inport
  y_t_dot : Inport  Port=2
  x_t_dot : Inport  Port=3
  phi_i_dot : Inport  Port=4
  Constant : Constant  Value=c
  Constant1 : Constant  Value=d
  IC : InitialCondition  Value=0
  IC1 : InitialCondition  Value=0
  Integrator : Integrator
  Integrator1 : Integrator
  MATLAB Function : MATLAB Function  TreatAsAtomicUnit=on
  Mux : Mux  Inputs=2
  Mux1 : Mux  Inputs=2
  To Workspace : ToWorkspace  VariableName=velocities_CG_i  SampleTime=-1
  To Workspace1 : ToWorkspace  VariableName=phi  SampleTime=-1
  phi_i : Outport
  phi_t : Outport  Port=2
  x_i_dot : Outport  Port=3
  y_i_dot : Outport  Port=4
  wires:
  MATLAB Function/1(x_i_cg_dot) -> Mux/1, x_i_dot/1
  Constant/1 -> MATLAB Function/7(c)
  Constant1/1 -> MATLAB Function/8(d)
  Integrator/1 -> IC1/1
  Integrator1/1 -> IC/1
  phi_t_dot/1 -> MATLAB Function/3(phi_t_dot), Integrator/1
  phi_i_dot/1 -> MATLAB Function/6(phi_i_dot), Integrator1/1
  x_t_dot/1 -> MATLAB Function/1(x_t_dot)
  y_t_dot/1 -> MATLAB Function/2(y_t_dot)
  IC/1 -> MATLAB Function/5(phi_i), Mux1/2, phi_i/1
  IC1/1 -> Mux1/1, phi_t/1, MATLAB Function/4(phi_t)
  MATLAB Function/2(y_i_cg_dot) -> Mux/2, y_i_dot/1
  Mux/1 -> To Workspace/1
  Mux1/1 -> To Workspace1/1

== system Coupled_Model_V2_C/EoMs/Aero Drag ==
  x_dot : Inport
  Gain : Gain  Gain=C_d
  Gain1 : Gain  Gain=0.5
  Gain2 : Gain  Gain=rho
  Gain3 : Gain  Gain=A
  Square : Math  Operator=square
  F_d : Outport
  wires:
  x_dot/1 -> Square/1
  Square/1 -> Gain/1
  Gain/1 -> Gain1/1
  Gain1/1 -> Gain2/1
  Gain2/1 -> Gain3/1
  Gain3/1 -> F_d/1

== system Coupled_Model_V2_C/Implement Wheel Torques/brake model ==
  brake_setpoint : Inport
  1_D brake toque table : Lookup_n-D  NumberOfTableDimensions=1  BreakpointsForDimension1=linspace(0,1, length(brake_torque))  Table=brake_torque  InternalRulePriority=Speed  RndMeth=Simplest
  brake_torque : Outport
  wires:
  1_D brake toque table/1 -> brake_torque/1  "brake torque"
  brake_setpoint/1 -> 1_D brake toque table/1  "[0:1]"

== system Coupled_Model_V2_C/Vehicle Slip Ratio/Long_tire_vel ==
  x_t_dot : Inport
  y_t_dot : Inport  Port=2
  phi_t_dot : Inport  Port=3
  delta_f : Inport  Port=4
  Constant : Constant  Value=a
  MATLAB Function : MATLAB Function  TreatAsAtomicUnit=on
  V_L_t_f : Outport
  V_L_t_r : Outport  Port=2
  wires:
  MATLAB Function/1(V_l_f) -> V_L_t_f/1
  MATLAB Function/2(V_l_r) -> V_L_t_r/1
  delta_f/1 -> MATLAB Function/1(delta_f)
  phi_t_dot/1 -> MATLAB Function/4(phi_dot)
  x_t_dot/1 -> MATLAB Function/2(x_dot)
  y_t_dot/1 -> MATLAB Function/3(y_dot)
  Constant/1 -> MATLAB Function/5(a)

== system Coupled_Model_V2_C/Vehicle Wheel Torques/brake model ==
  brake_setpoint : Inport
  1_D brake toque table : Lookup_n-D  NumberOfTableDimensions=1  BreakpointsForDimension1=linspace(0,1, length(brake_torque))  Table=brake_torque  InternalRulePriority=Speed  RndMeth=Simplest
  Gain : Gain  Gain=2*brake_bias
  Gain1 : Gain  Gain=2*(1-brake_bias)
  brake_torque_r : Outport
  brake_torque_f : Outport  Port=2
  wires:
  Gain/1 -> brake_torque_f/1
  Gain1/1 -> brake_torque_r/1
  1_D brake toque table/1 -> Gain/1, Gain1/1  "brake torque"
  brake_setpoint/1 -> 1_D brake toque table/1  "[0:1]"

== system Coupled_Model_V2_C/Vehicle Wheel Torques/engine model ==
  throttle setpoint : Inport
  omega_r : Inport  Port=2
  GR : Gain  Gain=gr
  Gain : Gain  Gain=1\gr
  Product : Product
  efficiency : Gain  Gain=drivetrain_e
  velocity to torque table : Lookup_n-D  NumberOfTableDimensions=1  BreakpointsForDimension1=torque_omega  Table=torque_curve  InternalRulePriority=Speed  RndMeth=Simplest
  engine_torque : Outport
  wires:
  efficiency/1 -> engine_torque/1
  GR/1 -> efficiency/1
  omega_r/1 -> Gain/1  "[rad/s]"
  Product/1 -> GR/1
  throttle setpoint/1 -> Product/1  "[0:1]"
  velocity to torque table/1 -> Product/2
  Gain/1 -> velocity to torque table/1  "engine speed"

== matlab function Coupled_Model_V2_C/Impliment Tire Model/MATLAB Function ==
  data: F_z input; mu input; c_sigma input; c_alpha input; F_y output; F_x output; sigma input; alpha input; peak_slip input; slip_coeff input
function [F_y, F_x]  = dugoff( F_z, mu, c_sigma, c_alpha, sigma, alpha, peak_slip, slip_coeff)
%Dugoff Model implemented

%add some feature where is slip angle is too high, it just slides at a
%constant frictional force.


lamda = (mu*F_z*(1+sigma))/(2*(((c_sigma*sigma)^2)+((c_alpha*tan(alpha))^2))^0.5);

if lamda < 1
    f_lamda = (2-lamda)*lamda;
else 
    f_lamda = 1;
end

F_x = c_sigma*(sigma/(1+sigma))*f_lamda;

if abs(alpha) > peak_slip
    if alpha >= 0
        F_y = F_z*slip_coeff;

    else
        F_y = -F_z*slip_coeff;

    end

else
    F_y = c_alpha*(tan(alpha)/(1+sigma))*f_lamda;
end

end

== matlab function Coupled_Model_V2_C/Velocity Transform/MATLAB Function ==
  data: x_t_dot input; x_i_cg_dot output; y_t_dot input; phi_t_dot input; phi_t input; phi_i input; phi_i_dot input; c input; d input; y_i_cg_dot output
function [x_i_cg_dot, y_i_cg_dot] = fcn(x_t_dot, y_t_dot, phi_t_dot, phi_t, phi_i, phi_i_dot, c, d)
%velocity transform

%convert frorm vehicle CG frame to global velocity at hitch (rotation 1)
x_global_H_dot = x_t_dot*cos(phi_t) - (y_t_dot - phi_t_dot*c)*sin(phi_t);
y_global_H_dot = x_t_dot*sin(phi_t) + (y_t_dot - phi_t_dot*c)*cos(phi_t);

%convert from global velocity at hitch to impliments frame (rotation 2)
x_i_hitch_dot = x_global_H_dot*cos(phi_i) + y_global_H_dot*sin(phi_i);
y_i_hitch_dot = -x_global_H_dot*sin(phi_i) + y_global_H_dot*cos(phi_i);

%convert from trailers pin to trailer cg
x_i_cg_dot = x_i_hitch_dot;
y_i_cg_dot = y_i_hitch_dot - phi_i_dot*d;


end

== matlab function Coupled_Model_V2_C/Force Transform/MATLAB Function ==
  data: phi_i input; F_t_x output; phi_t input; F_i_xh input; F_i_yh input; F_t_y output
function [F_t_x, F_t_y] = force_transform(phi_i, phi_t, F_i_xh, F_i_yh)

%convert to global coordinates
F_global_x = F_i_xh*cos(phi_i) + F_i_yh*sin(phi_i);
F_global_y = -F_i_xh*sin(phi_i) + F_i_yh*cos(phi_i);

%convert to implement frame
F_t_x = -F_global_x*cos(phi_t) + F_global_y*sin(phi_t);
F_t_y = -F_global_x*sin(phi_t) - F_global_y*cos(phi_t);

end

== matlab function Coupled_Model_V2_C/Impliment Slip Ratios/slip_ratio ==
  data: x_t_dot input; r input; sigma output; omega input; throttle input; trigger input
function sigma  = slip_ratio(x_t_dot, r, omega, throttle,  trigger)
%% Initialize output variables
sigma = 0;

%% calcualte tangential velocities
tangential_vel= r*omega; %[m/s]

%% calc slip ratio
if omega  < 0.01 && throttle ~= 0
    sigma = -0.001; %negative since so no positive torque  (aka resisting motion)
elseif trigger == 1 %prevent noise when at rest
    sigma = 0;
 elseif tangential_vel == 0 % keep this to prevent braking singularity
      sigma = 0;
elseif tangential_vel > x_t_dot %acceleration
    sigma = (tangential_vel-x_t_dot)/(tangential_vel);                   
elseif tangential_vel < x_t_dot %braking
    sigma = (tangential_vel - x_t_dot)/x_t_dot;
elseif tangential_vel == x_t_dot %must be true by definition
    sigma = 0;
end


end

== matlab function Coupled_Model_V2_C/INPUTS/MATLAB Function ==
  data: time input; out output; slope input; peak input; midpoint_t input
function out = fcn(time, slope, peak, midpoint_t)

out = peak./(1+exp(-4*(time-midpoint_t)/slope));

end

== matlab function Coupled_Model_V2_C/INPUTS/MATLAB Function2 ==
  data: time input; out output; slope input; peak input; midpoint_t input
function out = fcn(time, slope, peak, midpoint_t)

out = peak./(1+exp(-4*(time-midpoint_t)/slope));

end

== matlab function Coupled_Model_V2_C/INPUTS/set_zero ==
  data: in input; out output
function out = fcn(in)

if in < 0.0001
    out = 0;
elseif in == 0
    out = 0;
else 
    out = in;
end



end

== matlab function Coupled_Model_V2_C/INPUTS/MATLAB Function1 ==
  data: time input; out output; slope input; peak input; midpoint_t input
function out = fcn(time, slope, peak, midpoint_t)

out = peak./(1+exp(-4*(time-midpoint_t)/slope));

end

== matlab function Coupled_Model_V2_C/INPUTS/MATLAB Function3 ==
  data: time input; out output; slope input; peak input; midpoint_t input
function out = fcn(time, slope, peak, midpoint_t)

out = peak./(1+exp(-4*(time-midpoint_t)/slope));

end

== matlab function Coupled_Model_V2_C/Vehicle Tire Forces/MATLAB Function ==
  data: F_z_f input; F_y_f output; F_x_f output; F_z_r input; mu input; c_sigma input; c_alpha input; alpha_f input; sigma_f input; alpha_r input; sigma_r input; F_y_r output; F_x_r output
function [F_y_f, F_x_f, F_y_r, F_x_r]  = dugoff(F_z_f, F_z_r, mu, c_sigma, c_alpha, alpha_f, sigma_f, alpha_r, sigma_r)
%Dugoff Model implemented

%% calculate front tire forces
lamda_f = (mu*F_z_f*(1+sigma_f))/(2*(((c_sigma*sigma_f)^2)+((c_alpha*tan(alpha_f))^2))^0.5);

if lamda_f < 1
    f_lamda_f = (2-lamda_f)*lamda_f;
else %lamda_f >= 1
    f_lamda_f = 1;
end

F_x_f = c_sigma*(sigma_f/(1+sigma_f))*f_lamda_f;
F_y_f = c_alpha*(tan(alpha_f)/(1+sigma_f))*f_lamda_f;

%% calculate rear tire forces
lamda_r = (mu*F_z_r*(1+sigma_r))/(2*(((c_sigma*sigma_r)^2)+((c_alpha*tan(alpha_r))^2))^0.5);

if lamda_r < 1
    f_lamda_r = (2-lamda_r)*lamda_r;
else %lamda_r >= 1
    f_lamda_r = 1;
end

F_x_r = c_sigma*(sigma_r/(1+sigma_r))*f_lamda_r;
F_y_r = c_alpha*(tan(alpha_r)/(1+sigma_r))*f_lamda_r;


end

== matlab function Coupled_Model_V2_C/INPUTS/set_zero1 ==
  data: in input; out output
function out = fcn(in)

if in < 0.0001
    out = 0;
elseif in == 0
    out = 0;
else 
    out = in;
end



end

== matlab function Coupled_Model_V2_C/Vehicle Slsip Angles/MATLAB Function ==
  data: y_dot input; alpha_f output; x_dot input; phi_dot input; a input; b input; delta_f input; alpha_r output
function [alpha_f, alpha_r] = slip_angle(y_dot, x_dot, phi_dot, a, b, delta_f)
%calculates front and rear slip angles, units of [m] [rad/s] [m/s]
%equtions from 'VD and Control' textbook


if x_dot <= 0.01
    alpha_f = 0; %prevents singularity (cannot have slip at zero long. velocity)
    alpha_r = 0;
else
    alpha_f = delta_f - atan((y_dot + a*phi_dot)/x_dot);
    alpha_r = -atan((y_dot - b*phi_dot)/x_dot);
end


end

== matlab function Coupled_Model_V2_C/Vehicle Slip Ratio/slip_ratio ==
  data: V_l_f input; sigma_f output; V_l_r input; r input; omega_f input; omega_r input; sigma_r output; throttle input; trigger_f input; trigger_r input
function [sigma_f, sigma_r] = slip_ratio(V_l_f, V_l_r, r, omega_f, omega_r, throttle, trigger_f, trigger_r)
%% Initialize output variables
sigma_f = 0;
sigma_r = 0;

%% calcualte tangential velocities
tangential_vel_f = r*omega_f; %[m/s]
tangential_vel_r = r*omega_r; %[m/s]


%% calc front slip ratio
if omega_f ==0.0000  && throttle ~= 0
    sigma_f = -0.001; %negative since so no positive torque  (aka resisting motion)
elseif trigger_f == 1 %prevent noise when at rest
    sigma_f = 0;
 elseif tangential_vel_f == 0 % keep this to prevent braking singularity
      sigma_f = 0;
elseif tangential_vel_f > V_l_f %acceleration
    sigma_f = (tangential_vel_f-V_l_f)/(tangential_vel_f);                   
elseif tangential_vel_f < V_l_f %braking
    sigma_f = (tangential_vel_f - V_l_f)/V_l_f;
elseif tangential_vel_f == V_l_f %must be true by definition
    sigma_f = 0;
end

%% calc rear slip ratio
if  omega_r == 0  && throttle ~= 0 
    sigma_r = 0.001; %% tunable parameter 
elseif trigger_r == 1 %prevents odd fiedback
    sigma_r = 0;
elseif tangential_vel_r == 0
    sigma_r = 0;
elseif tangential_vel_r > V_l_r
    sigma_r = (tangential_vel_r-V_l_r)/(tangential_vel_r);
elseif tangential_vel_r < V_l_r
    sigma_r = (tangential_vel_r - V_l_r)/V_l_r;
elseif tangential_vel_r == V_l_r
    sigma_r = 0;
end

end

== matlab function Coupled_Model_V2_C/Vehicle Slip Ratio/Long_tire_vel/MATLAB Function ==
  data: delta_f input; V_l_f output; V_l_r output; x_dot input; y_dot input; phi_dot input; a input
function [V_l_f, V_l_r] = long_vel_tires(delta_f, x_dot, y_dot, phi_dot, a)
%% Calcualte tire/body frame velocites

%FRONT
V_y_f = y_dot + (a*phi_dot);
V_x_f = x_dot;
V_l_f = (V_y_f*sin(delta_f)) + (V_x_f*cos(delta_f));

%REAR
V_l_r = x_dot;


end

== matlab function Coupled_Model_V2_C/Vehicle Tire Forces/MATLAB Function1 ==
  data: Ft_y input; F_y output; Ft_x input; F_x output; delta input
function [F_y, F_x] = tire_force_transform(Ft_y, Ft_x, delta)

F_x = Ft_x*cos(delta) - Ft_y*sin(delta);

F_y = Ft_x*sin(delta) + Ft_y*cos(delta);

== matlab function Coupled_Model_V2_C/Vehicle Tire Forces/MATLAB Function2 ==
  data: Ft_y input; F_y output; Ft_x input; F_x output; delta input
function [F_y, F_x] = tire_force_transform(Ft_y, Ft_x, delta)

F_x = Ft_x*cos(delta) - Ft_y*sin(delta);

F_y = Ft_x*sin(delta) + Ft_y*cos(delta);

== matlab function Coupled_Model_V2_C/Impliment Slip Angle/MATLAB Function ==
  data: y_dot input; alpha output; x_dot input; phi_dot input; e input
function alpha  = slip_angle(y_dot, x_dot, phi_dot, e)
%calculates front and rear slip angles, units of [m] [rad/s] [m/s]
%equtions from 'VD and Control' textbook


if x_dot <= 0.01
    alpha = 0;
else
    alpha = -atan((y_dot - e*phi_dot)/x_dot);
end


end
